simulink model "inverse_pendulum_model"  (R2020a)
settings: Solver=VariableStepAuto  StartTime=0.0  StopTime=10  RelTol=1e-3
settings Model: Creator=MSI-PC  LastModifiedBy=MSI-PC

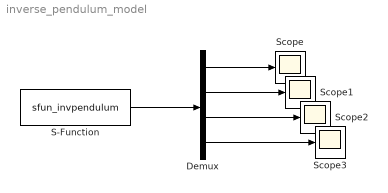
== system inverse_pendulum_model ==
  Demux : Demux
  S-Function : S-Function  FunctionName=sfun_invpendulum  SFunctionDeploymentMode=off  EnableBusSupport=off
  Scope{,1..3} (4 alike) : Scope
  wires:
  S-Function/1 -> Demux/1
  Demux/1 -> Scope/1
  Demux/2 -> Scope1/1
  Demux/3 -> Scope2/1
  Demux/4 -> Scope3/1
